simulink model "openloop"  (R2024b)
settings: Solver=VariableStepAuto  StartTime=0.0  StopTime=45  RelTol=1e-3
values from neighbouring files (symbols this model uses):
  atan_scale = 100    [threeDiskOscillator.m]
  b_1 = mean(ECP_values([6 7]))    [threeDiskOscillator.m]
  b_2 = mean(ECP_values([8 9]))    [threeDiskOscillator.m]
  b_3 = mean(ECP_values([10 11]))    [threeDiskOscillator.m]
  C = [  1 0 0 0 0 0 ... (first row only)    [threeDiskOscillator.m]
  G_r1u2_d = c2d(G_r1u2,T_s, 'tustin')    [threeDiskOscillator.m]
  G_r1y1_d = c2d(G_r1y1,T_s, 'tustin')    [threeDiskOscillator.m]
  G_r1y2_d = c2d(G_r1y2,T_s, 'tustin')    [threeDiskOscillator.m]
  G_r1y3_d = c2d(G_r1y3,T_s, 'tustin')    [threeDiskOscillator.m]
  G_r2y2_d = c2d(G_r2y2,T_s, 'tustin')    [threeDiskOscillator.m]
  G_r2y3_d = c2d(G_r2y3,T_s, 'tustin')    [threeDiskOscillator.m]
  J_1 = ECP_values(1)    [threeDiskOscillator.m]
  J_2 = ECP_values(2)    [threeDiskOscillator.m]
  J_3 = ECP_values(3)    [threeDiskOscillator.m]
  k_1 = ECP_values(4)    [threeDiskOscillator.m]
  k_2 = ECP_values(5)    [threeDiskOscillator.m]
  sigma_meas = 0.0093*eye(3)    [threeDiskOscillator.m]
  T_Cm = ECP_values(13)    [threeDiskOscillator.m]
  T_Cp = ECP_values(12)    [threeDiskOscillator.m]
  T_s = 0.004    [threeDiskOscillator.m]
  w_th = 0.75    [threeDiskOscillator.m]
  x_0 = [0;0;0;0;0;0]    [threeDiskOscillator.m]
settings Model: Creator=emma  LastModifiedBy=emma

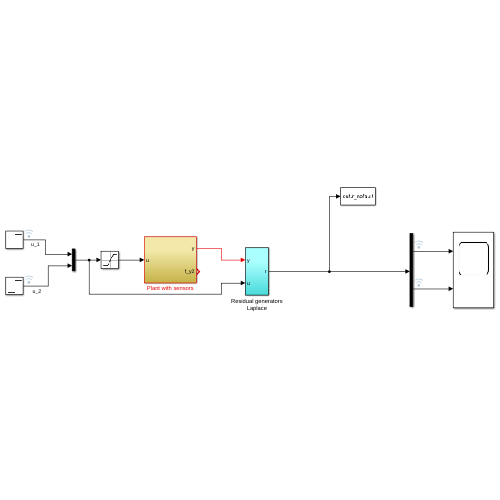
[thumbnail: Simulink's stored preview of the top-level diagram]
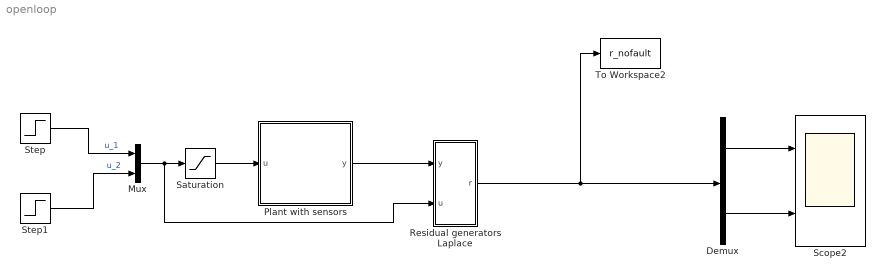
== system openloop ==
  Demux : Demux  Outputs=2
  Mux : Mux  Inputs=2
  Plant with sensors : Subsystem
  Residual generators Laplace : Subsystem
  Saturation : Saturate  UpperLimit=2  LowerLimit=-2
  Scope2 : Scope  NumInputPorts=2
  Step : Step  Time=5  SampleTime=0
  Step1 : Step  Time=10  After=2  SampleTime=0
  To Workspace2 : ToWorkspace  VariableName=r_nofault  SaveFormat=Timeseries  SampleTime=T_s
  wires:
  Plant with sensors/1(y) -> Residual generators Laplace/1(y)
  Mux/1 -> Saturation/1, Residual generators Laplace/2(u)
  Step/1 -> Mux/1  "u_1"
  Saturation/1 -> Plant with sensors/1(u)
  Residual generators Laplace/1(r) -> To Workspace2/1, Demux/1
  Step1/1 -> Mux/2  "u_2"
  Demux/1 -> Scope2/1
  Demux/2 -> Scope2/2

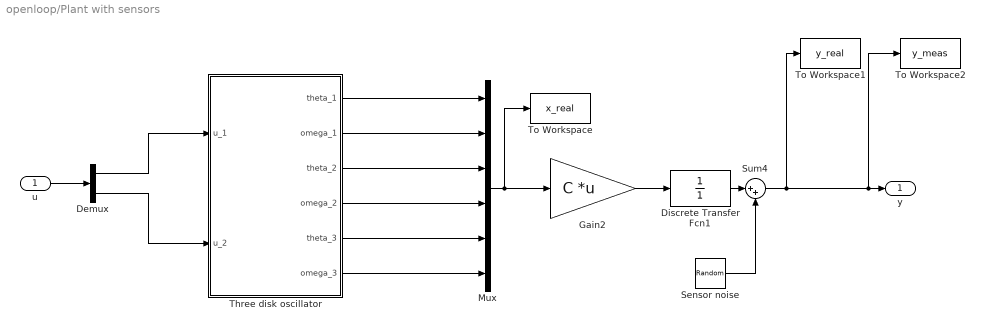
== system openloop/Plant with sensors ==
  u : Inport
  Demux : Demux  Outputs=2
  Discrete Transfer Fcn1 : DiscreteTransferFcn  Denominator=[1]  SampleTime=T_s
  Gain2 : Gain  Gain=C  Multiplication=Matrix(K*u) (u vector)
  Mux : Mux  Inputs=6
  Sensor noise : RandomNumber  Mean=zeros(3,1)  Variance=diag(sigma_meas^2)  SampleTime=T_s
  Sum4 : Sum  Inputs=|++
  Three disk oscillator : Subsystem
  To Workspace : ToWorkspace  VariableName=x_real  SaveFormat=Timeseries  SampleTime=T_s
  To Workspace1 : ToWorkspace  VariableName=y_real  SaveFormat=Timeseries  SampleTime=T_s
  To Workspace2 : ToWorkspace  VariableName=y_meas  SaveFormat=Timeseries  SampleTime=T_s
  y : Outport  VectorParamsAs1DForOutWhenUnconnected=off
  wires:
  u/1 -> Demux/1
  Three disk oscillator/2(omega_1) -> Mux/2
  Three disk oscillator/1(theta_1) -> Mux/1
  Three disk oscillator/4(omega_2) -> Mux/4
  Three disk oscillator/3(theta_2) -> Mux/3
  Gain2/1 -> Discrete Transfer Fcn1/1
  Three disk oscillator/6(omega_3) -> Mux/6
  Three disk oscillator/5(theta_3) -> Mux/5
  Sum4/1 -> To Workspace2/1, y/1, To Workspace1/1
  Demux/1 -> Three disk oscillator/1(u_1)
  Demux/2 -> Three disk oscillator/2(u_2)
  Mux/1 -> Gain2/1, To Workspace/1
  Discrete Transfer Fcn1/1 -> Sum4/1
  Sensor noise/1 -> Sum4/2

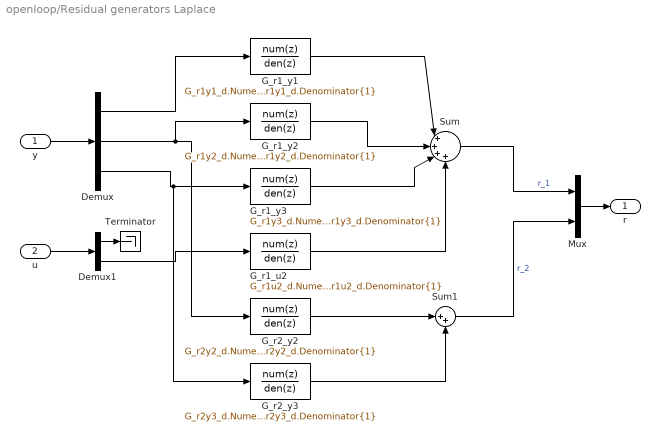
== system openloop/Residual generators Laplace ==
  y : Inport
  u : Inport  Port=2
  Demux : Demux  Outputs=3
  Demux1 : Demux  Outputs=2
  G_r1_u2 : DiscreteTransferFcn  Numerator=G_r1u2_d.Numerator{1}  Denominator=G_r1u2_d.Denominator{1}
  G_r1_y1 : DiscreteTransferFcn  Numerator=G_r1y1_d.Numerator{1}  Denominator=G_r1y1_d.Denominator{1}
  G_r1_y2 : DiscreteTransferFcn  Numerator=G_r1y2_d.Numerator{1}  Denominator=G_r1y2_d.Denominator{1}
  G_r1_y3 : DiscreteTransferFcn  Numerator=G_r1y3_d.Numerator{1}  Denominator=G_r1y3_d.Denominator{1}
  G_r2_y2 : DiscreteTransferFcn  Numerator=G_r2y2_d.Numerator{1}  Denominator=G_r2y2_d.Denominator{1}
  G_r2_y3 : DiscreteTransferFcn  Numerator=G_r2y3_d.Numerator{1}  Denominator=G_r2y3_d.Denominator{1}
  Mux : Mux  Inputs=2
  Sum : Sum  Inputs=|++++
  Sum1 : Sum  Inputs=|++
  Terminator : Terminator
  r : Outport  VectorParamsAs1DForOutWhenUnconnected=off
  wires:
  y/1 -> Demux/1
  Mux/1 -> r/1
  u/1 -> Demux1/1
  Sum/1 -> Mux/1  "r_1"
  Sum1/1 -> Mux/2  "r_2"
  Demux/1 -> G_r1_y1/1
  G_r1_y1/1 -> Sum/1
  Demux1/2 -> G_r1_u2/1
  G_r2_y2/1 -> Sum1/1
  G_r2_y3/1 -> Sum1/2
  G_r1_y2/1 -> Sum/2
  G_r1_y3/1 -> Sum/3
  G_r1_u2/1 -> Sum/4
  Demux/2 -> G_r2_y2/1, G_r1_y2/1
  Demux/3 -> G_r2_y3/1, G_r1_y3/1
  Demux1/1 -> Terminator/1

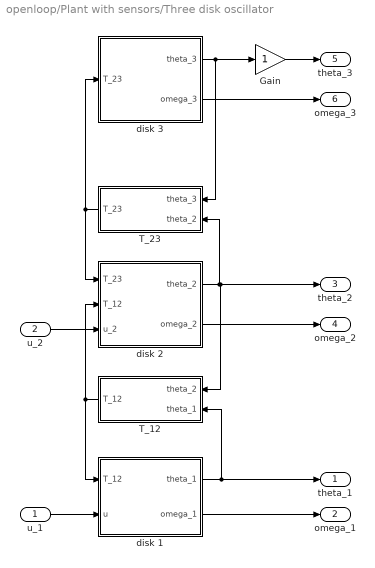
== system openloop/Plant with sensors/Three disk oscillator ==
  u_1 : Inport
  u_2 : Inport  Port=2
  Gain : Gain
  T_12 : Subsystem
  T_23 : Subsystem
  disk 1 : Subsystem
  disk 2 : Subsystem
  disk 3 : Subsystem
  theta_1 : Outport  VectorParamsAs1DForOutWhenUnconnected=off
  omega_1 : Outport  Port=2  VectorParamsAs1DForOutWhenUnconnected=off
  theta_2 : Outport  Port=3  VectorParamsAs1DForOutWhenUnconnected=off
  omega_2 : Outport  Port=4  VectorParamsAs1DForOutWhenUnconnected=off
  theta_3 : Outport  Port=5  VectorParamsAs1DForOutWhenUnconnected=off
  omega_3 : Outport  Port=6  VectorParamsAs1DForOutWhenUnconnected=off
  wires:
  T_23/1(T_23) -> disk 2/1(T_23), disk 3/1(T_23)
  disk 1/1(theta_1) -> T_12/2(theta_1), theta_1/1
  disk 2/1(theta_2) -> T_23/2(theta_2), theta_2/1, T_12/1(theta_2)
  T_12/1(T_12) -> disk 1/1(T_12), disk 2/2(T_12)
  disk 3/2(omega_3) -> omega_3/1
  disk 1/2(omega_1) -> omega_1/1
  disk 2/2(omega_2) -> omega_2/1
  u_1/1 -> disk 1/2(u)
  disk 3/1(theta_3) -> Gain/1, T_23/1(theta_3)
  Gain/1 -> theta_3/1
  u_2/1 -> disk 2/3(u_2)

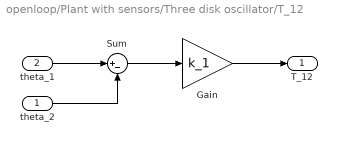
== system openloop/Plant with sensors/Three disk oscillator/T_12 ==
  theta_2 : Inport
  theta_1 : Inport  Port=2
  Gain : Gain  Gain=k_1
  Sum : Sum  Inputs=|+-
  T_12 : Outport  VectorParamsAs1DForOutWhenUnconnected=off
  wires:
  theta_2/1 -> Sum/2
  theta_1/1 -> Sum/1
  Sum/1 -> Gain/1
  Gain/1 -> T_12/1

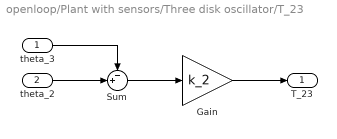
== system openloop/Plant with sensors/Three disk oscillator/T_23 ==
  theta_3 : Inport
  theta_2 : Inport  Port=2
  Gain : Gain  Gain=k_2
  Sum : Sum  Inputs=-+|
  T_23 : Outport  VectorParamsAs1DForOutWhenUnconnected=off
  wires:
  Gain/1 -> T_23/1
  Sum/1 -> Gain/1
  theta_3/1 -> Sum/1
  theta_2/1 -> Sum/2

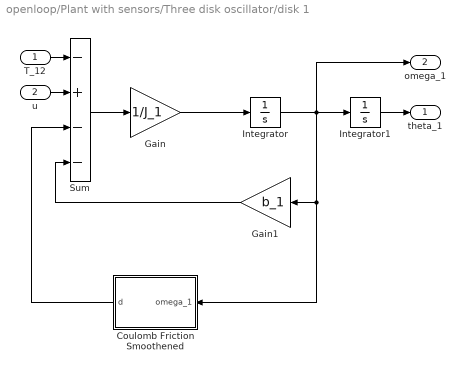
== system openloop/Plant with sensors/Three disk oscillator/disk 1 ==
  T_12 : Inport
  u : Inport  Port=2
  Coulomb Friction Smoothened : Subsystem
  Gain : Gain  Gain=1/J_1
  Gain1 : Gain  Gain=b_1
  Integrator : Integrator  InitialCondition=x_0(2)
  Integrator1 : Integrator  InitialCondition=x_0(1)
  Sum : Sum  Inputs=-+--
  theta_1 : Outport  VectorParamsAs1DForOutWhenUnconnected=off
  omega_1 : Outport  Port=2  VectorParamsAs1DForOutWhenUnconnected=off
  wires:
  Sum/1 -> Gain/1
  Integrator/1 -> Integrator1/1, omega_1/1, Coulomb Friction Smoothened/1(omega_1), Gain1/1
  Gain1/1 -> Sum/4
  Integrator1/1 -> theta_1/1
  T_12/1 -> Sum/1
  u/1 -> Sum/2
  Gain/1 -> Integrator/1
  Coulomb Friction Smoothened/1(d) -> Sum/3

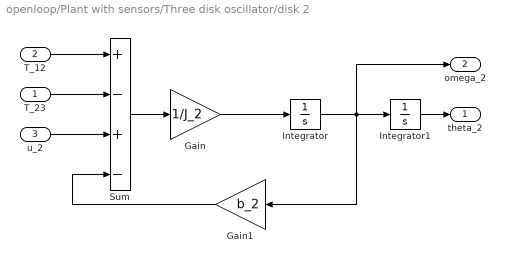
== system openloop/Plant with sensors/Three disk oscillator/disk 2 ==
  T_23 : Inport
  T_12 : Inport  Port=2
  u_2 : Inport  Port=3
  Gain : Gain  Gain=1/J_2
  Gain1 : Gain  Gain=b_2
  Integrator : Integrator  InitialCondition=x_0(4)
  Integrator1 : Integrator  InitialCondition=x_0(3)
  Sum : Sum  Inputs=+-+-
  theta_2 : Outport  VectorParamsAs1DForOutWhenUnconnected=off
  omega_2 : Outport  Port=2  VectorParamsAs1DForOutWhenUnconnected=off
  wires:
  T_23/1 -> Sum/2
  T_12/1 -> Sum/1
  Integrator1/1 -> theta_2/1
  Gain1/1 -> Sum/4
  Gain/1 -> Integrator/1
  Integrator/1 -> Integrator1/1, Gain1/1, omega_2/1
  Sum/1 -> Gain/1
  u_2/1 -> Sum/3

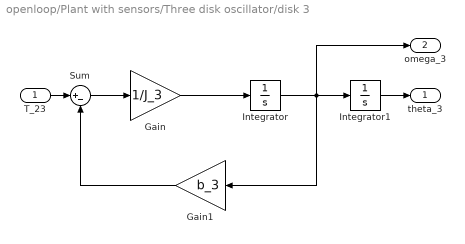
== system openloop/Plant with sensors/Three disk oscillator/disk 3 ==
  T_23 : Inport
  Gain : Gain  Gain=1/J_3
  Gain1 : Gain  Gain=b_3
  Integrator : Integrator  InitialCondition=x_0(6)
  Integrator1 : Integrator  InitialCondition=x_0(5)
  Sum : Sum  Inputs=|+-
  theta_3 : Outport  VectorParamsAs1DForOutWhenUnconnected=off
  omega_3 : Outport  Port=2  VectorParamsAs1DForOutWhenUnconnected=off
  wires:
  Sum/1 -> Gain/1
  Integrator/1 -> Integrator1/1, omega_3/1, Gain1/1
  Gain/1 -> Integrator/1
  Gain1/1 -> Sum/2
  Integrator1/1 -> theta_3/1
  T_23/1 -> Sum/1

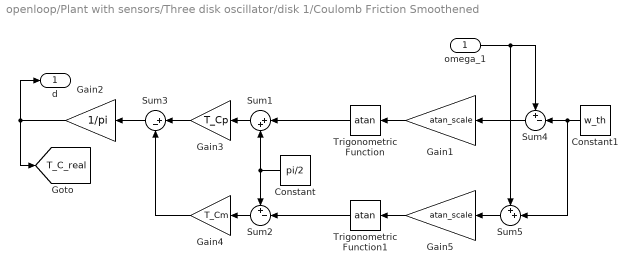
== system openloop/Plant with sensors/Three disk oscillator/disk 1/Coulomb Friction Smoothened ==
  omega_1 : Inport
  Constant : Constant  Value=pi/2
  Constant1 : Constant  Value=w_th
  Gain1 : Gain  Gain=atan_scale
  Gain2 : Gain  Gain=1/pi
  Gain3 : Gain  Gain=T_Cp
  Gain4 : Gain  Gain=T_Cm
  Gain5 : Gain  Gain=atan_scale
  Sum1 : Sum  Inputs=|++
  Sum2 : Sum  Inputs=+-|
  Sum3 : Sum  Inputs=|+-
  Sum4 : Sum  Inputs=+-|
  Sum5 : Sum  Inputs=++|
  Trigonometric Function : Trigonometry  Operator=atan
  Trigonometric Function1 : Trigonometry  Operator=atan
  d : Outport  VectorParamsAs1DForOutWhenUnconnected=off
  tag scope: T_C_real=global
  wires:
  Gain1/1 -> Trigonometric Function/1
  Sum1/1 -> Gain3/1
  Constant/1 -> Sum2/1, Sum1/2
  Sum2/1 -> Gain4/1
  Sum3/1 -> Gain2/1
  Trigonometric Function/1 -> Sum1/1
  Gain4/1 -> Sum3/2
  Gain2/1 -> [T_C_real], d/1
  omega_1/1 -> Sum5/1, Sum4/1
  Gain3/1 -> Sum3/1
  Sum4/1 -> Gain1/1
  Constant1/1 -> Sum5/2, Sum4/2
  Gain5/1 -> Trigonometric Function1/1
  Sum5/1 -> Gain5/1
  Trigonometric Function1/1 -> Sum2/2
